simulink model "freego_contact"  (Simulink 8.8)
settings: Solver=ode15s  StartTime=0.0  StopTime=30  MaxStep=0.04  MinStep=1e-10  RelTol=1e-3  EnableMultiTasking=on
model workspace (MATLAB code in the model file):
  | model = quadruped_robot();
undefined symbols (not defined in the file or in its folder): abad_InitAngle, Fpt, freego, gcontact, gcPosVel, hip_InitAngle, knee_InitAngle, quadruped_robot
libraries: simulink x9
settings Model: Creator=roy  LastModifiedBy=LZ
settings DataIOCC: LimitDataPoints=off
settings OptimizationCC: ExpressionDepthLimit=2147483647  InitFltsAndDblsToZero=on
settings DebuggingCC: SolverPrmCheckMsg=warning
settings GRTTargetCC: GeneratePreprocessorConditionals=Use local settings

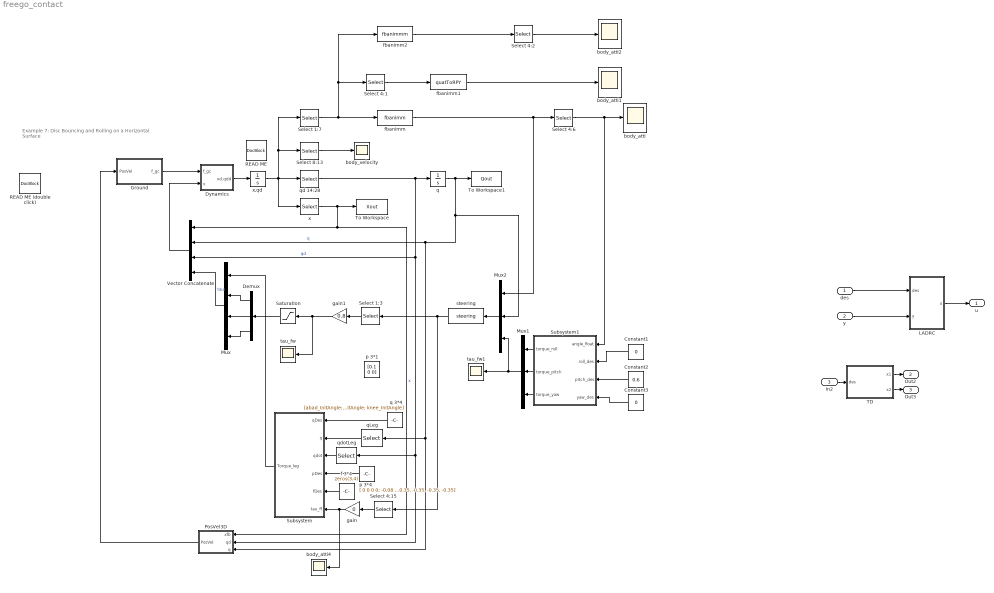
== system freego_contact ==
  note: Example 7: Disc Bouncing and Rolling
      | on a Horizontal Surface
  des : Inport
  y : Inport  Port=2
  In2 : Inport  Port=3
  Constant1 : Constant  Value=0
  Constant2 : Constant  Value=0.6
  Constant3 : Constant  Value=0
  Demux : Demux  Outputs=3
  Dynamics : Subsystem
  Ground : Subsystem
  LADRC : Subsystem
  Mux : Mux
  Mux1 : Mux  Inputs=3
  Mux2 : Mux  Inputs=3
  PosVel3D : Subsystem
  READ ME : simulink/Model-Wide Utilities/DocBlock  DocumentType=Text
      content=|
      | This subsystem builds upon the dynamics calculation in Example 4
      | (free-floating single rigid body).  The two new elements here are: a new
      | argument (f_gc) input to the dynamics calculation, and a new subsystem to
      | calculate the positions and velocities of the ground-contact points.
      |
      | Inside the "Dynamics" subsystem you will find that the floating-base state
      | vector, x, has been combined with the constant npoly and the matrix of
      | ground-contact forces, f_gc.  npoly is required as an argument to
      | rollingdisc.  The reason why it has to be supplied as an input like this
      | is because the executable expression in a "MATLAB Function" block does not
      | have access to the Simulink model's workspace (which is where npoly is
      | defined), so the symbol "npoly" cannot appear directly in this
      | expression.  f_gc is a 6x(npt) matrix, where npt is the number of points
      | defined in the rolling disc model, such that f_gc(:,i) is the spatial
      | force acting on point number i.  The "reshape" block converts it to a
      | column vector such that the first column of f_gc appears in the first six
      | elements, the second column in the next six elements, and so on.  The
      | function gcFD (appearing inside the "MATLAB Function" block) converts this
      | data into the cell-array format required by the f_ext arguments of the
      | dynamics functions, and calls FDfb to calculate the floating-base forward
      | dynamics of the rolling disc.
      |
      | Inside the "PosVel3D" subsystem, you will find the call to gcPosVel.  Once
      | again, npoly is supplied as a constant input, because it is needed as an
      | argument to rollingdisc but cannot appear explicitly in the executable
      | expression in the "MATLAB Function" block.  This function calculates a
      | 6x(npt) matrix such that column i contains the position (first three
      | elements) and velocity (last three elements) of point number i, both
      | expressed in base (body 0) coordinates.
      |
      | This dynamics subsystem can easily be adapted to fixed-base system models,
      | to floating-base models with more than one body, and to system models
      | based on planar arithmetic.  In the case of planar arithmetic, the
      | incoming f_gc is a 3x(npt) matrix whose columns are planar force vectors,
      | and the matrix calculated by gcPosVel is a 4x(npt) matrix containing two
      | 2D vectors in each column.  If vectors of joint position and velocity
      | variables (q and qd) are required instead of or in addition to x, then
      | these must be supplied as inputs to both gcFD and gcPosVel; so you will
      | have to add extra input ports to the blocks "Dynamics" and "PosVel3D".
  READ ME (double click) : simulink/Model-Wide Utilities/DocBlock  DocumentType=Text
  Saturation : Saturate  UpperLimit=3  LowerLimit=-3
  Select 1:3 : Selector  InputPortWidth=15  IndexOptions=Index vector (dialog)  Indices=[1:3]  OutputSizes=1
  Select 1:7 : Selector  InputPortWidth=13+15  IndexOptions=Index vector (dialog)  Indices=[1:7]  OutputSizes=1
  Select 4:1 : Selector  InputPortWidth=7  IndexOptions=Index vector (dialog)  Indices=[1:4]  OutputSizes=1
  Select 4:15 : Selector  InputPortWidth=15  IndexOptions=Index vector (dialog)  Indices=[4:15]  OutputSizes=1
  Select 4:2 : Selector  InputPortWidth=6  IndexOptions=Index vector (dialog)  Indices=[4:6]  OutputSizes=1
  Select 4:6 : Selector  InputPortWidth=6  IndexOptions=Index vector (dialog)  Indices=[4:6]  OutputSizes=1
  Select 8:13 : Selector  InputPortWidth=13+15  IndexOptions=Index vector (dialog)  Indices=[8 9 10 11 12 13]  OutputSizes=1
  Subsystem : Subsystem
  Subsystem1 : Subsystem
  TD : Subsystem
  To Workspace : ToWorkspace  VariableName=Xout  SampleTime=-1
  To Workspace1 : ToWorkspace  VariableName=Qout  SampleTime=-1
  Vector Concatenate : Concatenate  NumInputs=4
  body_atti{,1..2,4} (4 alike) : Scope
  body_velocity : Scope
  f 3*4 : Constant  Value=zeros(3,4)
  fbanimm : MATLABFcn  MATLABFcn=fbanimm  OutputDimensions=6
  fbanimm1 : MATLABFcn  MATLABFcn=quatToRPY  OutputDimensions=3
  fbanimm2 : MATLABFcn  MATLABFcn=fbanimmm  OutputDimensions=6
  gain : Gain  Gain=0
  gain1 : Gain  Gain=0.8
  p 3*1 : Constant  Value=[0.1 0 0]
  p 3*4 : Constant  Value=[ 0 0 0 0; -0.08 0.08 -0.08 0.08; -0.35, -0.35, -0.35, -0.35]
  q : Integrator  InitialCondition=[freego.q_init]'
  q 3*4 : Constant  Value=[abad_InitAngle; hip_InitAngle; knee_InitAngle]
  qLeg : Selector  InputPortWidth=15  IndexOptions=Index vector (dialog)  Indices=[1:12]  OutputSizes=1
  qd 14:28 : Selector  InputPortWidth=13+15  IndexOptions=Index vector (dialog)  Indices=[14:13+15]  OutputSizes=1
  qdotLeg : Selector  InputPortWidth=15  IndexOptions=Index vector (dialog)  Indices=[1:12]  OutputSizes=1
  steering : MATLABFcn  MATLABFcn=steering  OutputDimensions=15  Output1D=off
  tau_fw : Scope
  tau_fw1 : Scope
  x : Selector  InputPortWidth=13+15  IndexOptions=Index vector (dialog)  Indices=[1:13]  OutputSizes=1
  x,qd : Integrator  InitialCondition=[freego.QuatBody, freego.COMLocation, zeros(1,6), zeros(1,15)]'
  u : Outport
  Out2 : Outport  Port=2
  Out3 : Outport  Port=3
  wires:
  PosVel3D/1(PosVel) -> Ground/1(PosVel)
  Dynamics/1(xd,qdd) -> x,qd/1
  x,qd/1 -> x/1, qd 14:28/1, Select 1:7/1, Select 8:13/1
  Select 8:13/1 -> body_velocity/1
  qd 14:28/1 -> q/1, PosVel3D/2(qd), qdotLeg/1, Vector Concatenate/3  "qd"
  q/1 -> To Workspace1/1, Mux2/2, Vector Concatenate/2, PosVel3D/3(q), qLeg/1  "q"
  x/1 -> To Workspace/1, Vector Concatenate/1, PosVel3D/1(xfb)  "x"
  Vector Concatenate/1 -> Dynamics/2(x)
  Ground/1(f_gc) -> Dynamics/1(f_gc)
  Mux/1 -> Vector Concatenate/4  "tau"
  des/1 -> LADRC/1(des)
  y/1 -> LADRC/2(y)
  LADRC/1(u) -> u/1
  In2/1 -> TD/1(des)
  TD/2(x2) -> Out3/1
  TD/1(x1) -> Out2/1
  Demux/1 -> Mux/2
  q 3*4/1 -> Subsystem/1(qDes)
  Subsystem/1(Torque_leg) -> Mux/1
  p 3*4/1 -> Subsystem/4(pDes)
  f 3*4/1 -> Subsystem/5(fDes)
  qLeg/1 -> Subsystem/2(q)
  qdotLeg/1 -> Subsystem/3(qdot)
  Demux/3 -> Mux/4
  Select 1:7/1 -> fbanimm2/1, Select 4:1/1, fbanimm/1
  fbanimm/1 -> Mux2/1, Select 4:6/1
  Select 4:6/1 -> body_atti/1, Subsystem1/1(angle_float)
  Constant2/1 -> Subsystem1/3(pitch_des)
  Subsystem1/1(torque_roll) -> Mux1/1
  Subsystem1/2(torque_pitch) -> Mux1/2
  Subsystem1/3(torque_yaw) -> Mux1/3
  Mux2/1 -> steering/1
  Mux1/1 -> Mux2/3, tau_fw1/1
  steering/1 -> Select 4:15/1, Select 1:3/1
  Demux/2 -> Mux/3
  gain1/1 -> tau_fw/1, Saturation/1
  Select 4:15/1 -> gain/1
  Constant1/1 -> Subsystem1/2(roll_des)
  Constant3/1 -> Subsystem1/4(yaw_des)
  gain/1 -> Subsystem/6(tau_ff), body_atti4/1
  Saturation/1 -> Demux/1
  Select 4:1/1 -> fbanimm1/1
  fbanimm1/1 -> body_atti1/1
  fbanimm2/1 -> Select 4:2/1
  Select 4:2/1 -> body_atti2/1
  Select 1:3/1 -> gain1/1

== system freego_contact/Dynamics ==
  f_gc : Inport
  x : Inport  Port=2
  Quadruped_robot  Dynamics : MATLABFcn  MATLABFcn=gcFD( quadruped_robot, @FDfb, u )  OutputDimensions=[13+15 1]  OutputSignalType=real  Output1D=off
  Reshape : Reshape  OutputDimensionality=Column vector (2-D)
  Vector Concatenate : Concatenate
  xd,qdd : Outport
  wires:
  Vector Concatenate/1 -> Quadruped_robot  Dynamics/1
  Quadruped_robot  Dynamics/1 -> xd,qdd/1
  f_gc/1 -> Reshape/1
  x/1 -> Vector Concatenate/1
  Reshape/1 -> Vector Concatenate/2

== system freego_contact/Ground ==
  PosVel : Inport
  3D Ground Contact : Subsystem  mask(3D Nonlinear Ground Contact with Friction){K=1e6, D=2000, mu=0.1, np=16}
      mask prompts: K "Stiffness (K)"; D "Damping (D)"; mu "Coefficient of Friction (mu)"; np "Number of Contact Points"
      mask help:
      | Given two 3xnp arrays containing contact-point positions and
      | velocities, calculate the 3xnp array of ground-reaction forces
      | acting on those points. Also calculate 1xnp boolean vectors
      | in_ctact (true if normal force >0) and sticking (true if inside
      | or on boundary of friction cone).  Zero-crossing detection is
      | enabled at both make/break contact and stick/slip transitions.
  READ ME : simulink/Model-Wide Utilities/DocBlock  DocumentType=Text
  Terminator : Terminator
  Terminator1 : Terminator
  convert 3D to spatial forces : Subsystem
  select pos : Selector  NumberOfDimensions=2  InputPortWidth=3  IndexOptions=Index vector (dialog),Select all  Indices=[1 2 3],1  OutputSizes=1,1
  select vel : Selector  NumberOfDimensions=2  InputPortWidth=3  IndexOptions=Index vector (dialog),Select all  Indices=[4 5 6],1  OutputSizes=1,1
  f_gc : Outport
  wires:
  PosVel/1 -> select pos/1, select vel/1
  select pos/1 -> convert 3D to spatial forces/1(pos), 3D Ground Contact/1(pos)
  convert 3D to spatial forces/1(force6D) -> f_gc/1
  select vel/1 -> 3D Ground Contact/2(vel)
  3D Ground Contact/1(force) -> convert 3D to spatial forces/2(force3D)
  3D Ground Contact/2(in_ctact) -> Terminator/1
  3D Ground Contact/3(sticking) -> Terminator1/1

== system freego_contact/LADRC ==
  des : Inport
  y : Inport  Port=2
  1/b0 : Gain
  LESO3 : Subsystem
  PID Controller : simulink/Continuous/PID Controller  Controller=PID  TimeDomain=Continuous-time  SampleTime=-1  IntegratorMethod=Forward Euler  FilterMethod=Forward Euler  Form=Parallel  UseFilter=on  ControllerParametersSource=internal  P=10  I=0.01  D=1  N=100  InitialConditionSource=internal  InitialConditionForIntegrator=0  InitialConditionForFilter=0  ExternalReset=none  LimitOutput=off  UpperSaturationLimit=inf  LowerSaturationLimit=-inf  LinearizeAsGain=on  AntiWindupMode=none  Kb=1  TrackingMode=off  Kt=1  PParamMin=[]  PParamMax=[]  IParamMin=[]  IParamMax=[]  DParamMin=[]  DParamMax=[]  NParamMin=[]  NParamMax=[]  KbParamMin=[]  KbParamMax=[]  KtParamMin=[]  KtParamMax=[]  POutMin=[]  POutMax=[]  IOutMin=[]  IOutMax=[]  DOutMin=[]  DOutMax=[]  NOutMin=[]  NOutMax=[]  KbOutMin=[]  KbOutMax=[]  KtOutMin=[]  KtOutMax=[]  IntegratorOutMin=[]  IntegratorOutMax=[]  FilterOutMin=[]  FilterOutMax=[]  SumOutMin=[]  SumOutMax=[]  SumI1OutMin=[]  SumI1OutMax=[]  SumI2OutMin=[]  SumI2OutMax=[]  SumI3OutMin=[]  SumI3OutMax=[]  SumDOutMin=[]  SumDOutMax=[]  SaturationOutMin=[]  SaturationOutMax=[]  IntegratorContinuousStateAttributes=''  IntegratorStateMustResolveToSignalObject=off  IntegratorRTWStateStorageClass=Auto  FilterContinuousStateAttributes=''  FilterStateMustResolveToSignalObject=off  FilterRTWStateStorageClass=Auto  DifferentiatorICPrevScaledInput=0  DifferentiatorOutMin=[]  DifferentiatorOutMax=[]
  PID Controller1 : simulink/Continuous/PID Controller  Controller=PID  TimeDomain=Continuous-time  SampleTime=-1  IntegratorMethod=Forward Euler  FilterMethod=Forward Euler  Form=Parallel  UseFilter=on  ControllerParametersSource=internal  P=10  I=0.01  D=1  N=100  InitialConditionSource=internal  InitialConditionForIntegrator=0  InitialConditionForFilter=0  ExternalReset=none  LimitOutput=off  UpperSaturationLimit=inf  LowerSaturationLimit=-inf  LinearizeAsGain=on  AntiWindupMode=none  Kb=1  TrackingMode=off  Kt=1  PParamMin=[]  PParamMax=[]  IParamMin=[]  IParamMax=[]  DParamMin=[]  DParamMax=[]  NParamMin=[]  NParamMax=[]  KbParamMin=[]  KbParamMax=[]  KtParamMin=[]  KtParamMax=[]  POutMin=[]  POutMax=[]  IOutMin=[]  IOutMax=[]  DOutMin=[]  DOutMax=[]  NOutMin=[]  NOutMax=[]  KbOutMin=[]  KbOutMax=[]  KtOutMin=[]  KtOutMax=[]  IntegratorOutMin=[]  IntegratorOutMax=[]  FilterOutMin=[]  FilterOutMax=[]  SumOutMin=[]  SumOutMax=[]  SumI1OutMin=[]  SumI1OutMax=[]  SumI2OutMin=[]  SumI2OutMax=[]  SumI3OutMin=[]  SumI3OutMax=[]  SumDOutMin=[]  SumDOutMax=[]  SaturationOutMin=[]  SaturationOutMax=[]  IntegratorContinuousStateAttributes=''  IntegratorStateMustResolveToSignalObject=off  IntegratorRTWStateStorageClass=Auto  FilterContinuousStateAttributes=''  FilterStateMustResolveToSignalObject=off  FilterRTWStateStorageClass=Auto  DifferentiatorICPrevScaledInput=0  DifferentiatorOutMin=[]  DifferentiatorOutMax=[]
  Sum1 : Sum  Inputs=|+-
  Sum2 : Sum  Inputs=|+-
  Sum3 : Sum  Inputs=+|+
  Sum4 : Sum  Inputs=|+-
  "TD3 " : Subsystem
  b0 : Gain
  u : Outport
  wires:
  des/1 -> "TD3 "/1(des)
  Sum3/1 -> Sum4/1
  1/b0/1 -> Sum4/2
  PID Controller1/1 -> Sum3/2
  y/1 -> LESO3/1(y)
  Sum2/1 -> PID Controller1/1
  LESO3/3(z3) -> 1/b0/1
  PID Controller/1 -> Sum3/1
  "TD3 "/2(x2) -> Sum2/1
  LESO3/2(z2) -> Sum2/2
  "TD3 "/1(x1) -> Sum1/1
  Sum1/1 -> PID Controller/1
  b0/1 -> LESO3/2(b0u)
  LESO3/1(z1) -> Sum1/2
  Sum4/1 -> u/1, b0/1

== system freego_contact/PosVel3D ==
  note: The constant supplies the
      | argument for rollingdisc
  xfb : Inport
  qd : Inport  Port=2
  q : Inport  Port=3
  Vector Concatenate1 : Concatenate  NumInputs=3
  gcPosVel : MATLABFcn  MATLABFcn=gcPosVel( quadruped_robot(), u(1:13), u(14:28), u(29:43))  OutputDimensions=[6 16]  OutputSignalType=real  Output1D=off
  PosVel : Outport
  wires:
  gcPosVel/1 -> PosVel/1
  Vector Concatenate1/1 -> gcPosVel/1
  q/1 -> Vector Concatenate1/2
  xfb/1 -> Vector Concatenate1/1
  qd/1 -> Vector Concatenate1/3

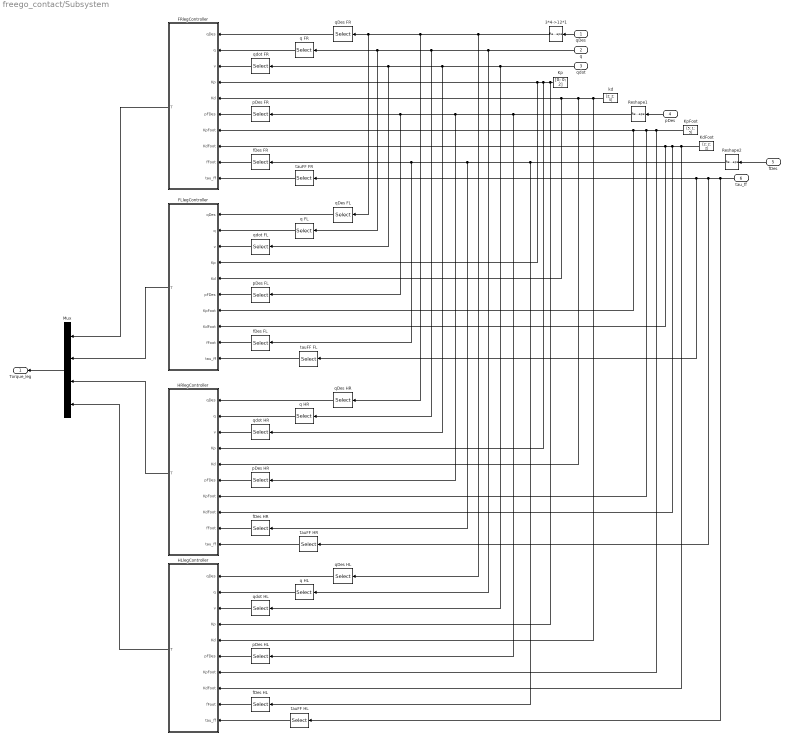
== system freego_contact/Subsystem ==
  qDes : Inport
  q : Inport  Port=2
  qdot : Inport  Port=3
  pDes : Inport  Port=4
  fDes : Inport  Port=5
  tau_ff : Inport  Port=6
  3*4->12*1 : Reshape  OutputDimensionality=Column vector (2-D)
  FLlegController : Subsystem
  FRlegController : Subsystem
  HLlegController : Subsystem
  HRlegController : Subsystem
  KdFoot : Constant  Value=[2; 2; 2]
  Kp : Constant  Value=[0; 0; 2]
  KpFoot : Constant  Value=[5; 1; 5]
  Mux : Mux
  Reshape1 : Reshape  OutputDimensionality=Column vector (2-D)
  Reshape2 : Reshape  OutputDimensionality=Column vector (2-D)
  fDes FL : Selector  InputPortWidth=12  IndexOptions=Index vector (dialog)  Indices=[4:6]  OutputSizes=1
  fDes FR : Selector  InputPortWidth=12  IndexOptions=Index vector (dialog)  Indices=[1:3]  OutputSizes=1
  fDes HL : Selector  InputPortWidth=12  IndexOptions=Index vector (dialog)  Indices=[10:12]  OutputSizes=1
  fDes HR : Selector  InputPortWidth=12  IndexOptions=Index vector (dialog)  Indices=[7:9]  OutputSizes=1
  kd : Constant  Value=[2; 2; 5]
  pDes FL : Selector  InputPortWidth=12  IndexOptions=Index vector (dialog)  Indices=[4:6]  OutputSizes=1
  pDes FR : Selector  InputPortWidth=12  IndexOptions=Index vector (dialog)  Indices=[1:3]  OutputSizes=1
  pDes HL : Selector  InputPortWidth=12  IndexOptions=Index vector (dialog)  Indices=[10:12]  OutputSizes=1
  pDes HR : Selector  InputPortWidth=12  IndexOptions=Index vector (dialog)  Indices=[7:9]  OutputSizes=1
  q FL : Selector  InputPortWidth=12  IndexOptions=Index vector (dialog)  Indices=[4:6]  OutputSizes=1
  q FR : Selector  InputPortWidth=12  IndexOptions=Index vector (dialog)  Indices=[1:3]  OutputSizes=1
  q HL : Selector  InputPortWidth=12  IndexOptions=Index vector (dialog)  Indices=[10:12]  OutputSizes=1
  q HR : Selector  InputPortWidth=12  IndexOptions=Index vector (dialog)  Indices=[7:9]  OutputSizes=1
  qDes FL : Selector  InputPortWidth=12  IndexOptions=Index vector (dialog)  Indices=[4:6]  OutputSizes=1
  qDes FR : Selector  InputPortWidth=12  IndexOptions=Index vector (dialog)  Indices=[1:3]  OutputSizes=1
  qDes HL : Selector  InputPortWidth=12  IndexOptions=Index vector (dialog)  Indices=[10:12]  OutputSizes=1
  qDes HR : Selector  InputPortWidth=12  IndexOptions=Index vector (dialog)  Indices=[7:9]  OutputSizes=1
  qdot FL : Selector  InputPortWidth=12  IndexOptions=Index vector (dialog)  Indices=[4:6]  OutputSizes=1
  qdot FR : Selector  InputPortWidth=12  IndexOptions=Index vector (dialog)  Indices=[1:3]  OutputSizes=1
  qdot HL : Selector  InputPortWidth=12  IndexOptions=Index vector (dialog)  Indices=[10:12]  OutputSizes=1
  qdot HR : Selector  InputPortWidth=12  IndexOptions=Index vector (dialog)  Indices=[7:9]  OutputSizes=1
  tauFF FL : Selector  InputPortWidth=12  IndexOptions=Index vector (dialog)  Indices=[4:6]  OutputSizes=1
  tauFF FR : Selector  InputPortWidth=12  IndexOptions=Index vector (dialog)  Indices=[1:3]  OutputSizes=1
  tauFF HL : Selector  InputPortWidth=12  IndexOptions=Index vector (dialog)  Indices=[10:12]  OutputSizes=1
  tauFF HR : Selector  InputPortWidth=12  IndexOptions=Index vector (dialog)  Indices=[7:9]  OutputSizes=1
  Torque_leg : Outport
  wires:
  q FR/1 -> FRlegController/2(q)
  qDes/1 -> 3*4->12*1/1
  pDes/1 -> Reshape1/1
  qdot/1 -> qdot HR/1, qdot FL/1, qdot FR/1, qdot HL/1
  qdot FR/1 -> FRlegController/3(v)
  q FL/1 -> FLlegController/2(q)
  kd/1 -> HLlegController/5(Kd), HRlegController/5(Kd), FLlegController/5(Kd), FRlegController/5(Kd)
  KpFoot/1 -> FRlegController/7(KpFoot), FLlegController/7(KpFoot), HRlegController/7(KpFoot), HLlegController/7(KpFoot)
  qDes FL/1 -> FLlegController/1(qDes)
  pDes FL/1 -> FLlegController/6(pFDes)
  q/1 -> q HR/1, q FL/1, q FR/1, q HL/1
  qdot FL/1 -> FLlegController/3(v)
  qDes FR/1 -> FRlegController/1(qDes)
  pDes FR/1 -> FRlegController/6(pFDes)
  3*4->12*1/1 -> qDes HR/1, qDes FL/1, qDes FR/1, qDes HL/1
  Reshape1/1 -> pDes HR/1, pDes FL/1, pDes FR/1, pDes HL/1
  q HR/1 -> HRlegController/2(q)
  qDes HR/1 -> HRlegController/1(qDes)
  pDes HR/1 -> HRlegController/6(pFDes)
  qdot HR/1 -> HRlegController/3(v)
  q HL/1 -> HLlegController/2(q)
  Kp/1 -> HLlegController/4(Kp), HRlegController/4(Kp), FLlegController/4(Kp), FRlegController/4(Kp)
  KdFoot/1 -> FRlegController/8(KdFoot), FLlegController/8(KdFoot), HRlegController/8(KdFoot), HLlegController/8(KdFoot)
  Reshape2/1 -> fDes HL/1, fDes HR/1, fDes FL/1, fDes FR/1
  qDes HL/1 -> HLlegController/1(qDes)
  pDes HL/1 -> HLlegController/6(pFDes)
  qdot HL/1 -> HLlegController/3(v)
  Mux/1 -> Torque_leg/1
  FRlegController/1(T) -> Mux/1
  FLlegController/1(T) -> Mux/2
  HRlegController/1(T) -> Mux/3
  HLlegController/1(T) -> Mux/4
  fDes/1 -> Reshape2/1
  fDes FR/1 -> FRlegController/9(fFoot)
  fDes FL/1 -> FLlegController/9(fFoot)
  fDes HR/1 -> HRlegController/9(fFoot)
  fDes HL/1 -> HLlegController/9(fFoot)
  tauFF FL/1 -> FLlegController/10(tau_ff)
  tauFF HR/1 -> HRlegController/10(tau_ff)
  tauFF HL/1 -> HLlegController/10(tau_ff)
  tauFF FR/1 -> FRlegController/10(tau_ff)
  tau_ff/1 -> tauFF HL/1, tauFF HR/1, tauFF FL/1, tauFF FR/1

== system freego_contact/Subsystem1 ==
  angle_float : Inport
  roll_des : Inport  Port=2
  pitch_des : Inport  Port=3
  yaw_des : Inport  Port=4
  Demux : Demux  Outputs=3
  LADRC_Pitch : Subsystem
  LADRC_Roll : Subsystem
  LADRC_Yaw : Subsystem
  p : Gain  Gain=0
  p1 : Gain  Gain=-1
  p2 : Gain  Gain=0
  torque_roll : Outport
  torque_pitch : Outport  Port=2
  torque_yaw : Outport  Port=3
  wires:
  LADRC_Yaw/1(u) -> p2/1
  yaw_des/1 -> LADRC_Yaw/1(des)
  pitch_des/1 -> LADRC_Pitch/1(des)
  LADRC_Pitch/1(u) -> p1/1
  angle_float/1 -> Demux/1
  p/1 -> torque_roll/1
  roll_des/1 -> LADRC_Roll/1(des)
  LADRC_Roll/1(u) -> p/1
  Demux/2 -> LADRC_Pitch/2(y)
  Demux/1 -> LADRC_Roll/2(y)
  Demux/3 -> LADRC_Yaw/2(y)
  p1/1 -> torque_pitch/1
  p2/1 -> torque_yaw/1

== system freego_contact/TD ==
  des : Inport
  MATLAB Function1 : MATLAB Function  TreatAsAtomicUnit=on
  Product : Product
  Product1 : Product
  Sum : Sum  Inputs=+-|
  h : Constant
  r : Constant  Value=10000000000000000000000000
  sx1 : Integrator
  sx2 : Integrator
  x1 : Outport
  x2 : Outport  Port=2
  wires:
  sx2/1 -> MATLAB Function1/2(x2), x2/1, Product1/1
  h/1 -> MATLAB Function1/4(h), Product/2, Product1/2  "h"
  Product/1 -> sx2/1
  MATLAB Function1/1(fh) -> Product/1
  sx1/1 -> Sum/1, x1/1
  r/1 -> MATLAB Function1/3(r)
  Product1/1 -> sx1/1
  Sum/1 -> MATLAB Function1/1(x1)
  des/1 -> Sum/2

== system freego_contact/Ground/3D Ground Contact ==
  pos : Inport
  vel : Inport  Port=2
  Compare To Constant : simulink/Logic and Bit Operations/Compare To Constant  relop=<=  const=1  OutDataTypeStr=boolean
  Compare To Zero : simulink/Logic and Bit Operations/Compare To Zero  relop=>  OutDataTypeStr=boolean
  K,D,mu : Constant  Value=[ [K; D; mu] zeros(3,np-1) ]  VectorParams1D=off
  READ ME : simulink/Model-Wide Utilities/DocBlock  DocumentType=Text
      content=|
      | The constant block supplies the parameters K, D and mu to the function
      | gcontact.  This is necessary because K, D and mu are defined in the
      | workspace of this particular masked subsystem, but the executable
      | expression in the "MATLAB Function" block does not have access to this
      | workspace, so the symbols K, D and mu cannot appear directly in the
      | executable expression.
      |
      | The ">0" block and the "<=1" block both have zero-crossing enabled.  The
      | former detects transitions between contact and non-contact, whereas the
      | latter detects transitions between sticking (due to friction) and
      | slipping.  A point can be sticking only if it is also in contact.  A
      | zero-crossing event occurs whenever any one point makes a transition.
      |
      | The state variable, u, is a 2x(np) matrix containing the horizontal
      | component of the local ground deformation for each point.  This quantity
      | is used to calculate the tangential (i.e., frictional) component of the
      | ground reaction force.
      |
      | When a point loses contact, its associated state variable, u(:,i), decays
      | to zero with a time constant of D/K.  If this ratio is small then the
      | corresponding differential equation is fast, and it is necessary to use
      | small integration time steps.  For example, if K=1e6 and D=2000 then
      | D/K=0.002 and u(:,i) decays in proportion to exp(-500t).  Increasing K
      | makes the surface stiffer, and decreasing D/K makes it bouncier, but the
      | latter also makes the post-contact recovery faster.  The degree of
      | bounciness depends on the mass of the impacting body: a heavier body will
      | bounce more.
      |
      | To adapt this subsystem to work in 2D, the only things that change are the
      | row dimensions of various matrices.  You will have to alter the row
      | selections in the executable expression in the "MATLAB Function" block,
      | and also the dimensions of its output matrix, and you will have to change
      | the row selections in the various "select" blocks.
      |
      | For more information, see "The Simulink Ground Contact Model" in the
      | spatial_v2 documentation directory.
  Vector Concatenate : Concatenate  NumInputs=4  Mode=Multidimensional array
  gcontact : MATLABFcn  MATLABFcn=gcontact( u(1,1), u(2,1), u(3,1), u(4:6,:), u(7:9,:), u(10:11,:) )  OutputDimensions=[6 np]  OutputSignalType=real  Output1D=off
  select fcone : Selector  NumberOfDimensions=2  InputPortWidth=3  IndexOptions=Index vector (dialog),Select all  Indices=[6],1  OutputSizes=1,1
  select force : Selector  NumberOfDimensions=2  InputPortWidth=3  IndexOptions=Index vector (dialog),Select all  Indices=[1 2 3],1  OutputSizes=1,1
  select fz : Selector  NumberOfDimensions=2  InputPortWidth=3  IndexOptions=Index vector (dialog),Select all  Indices=[3],1  OutputSizes=1,1
  select ud : Selector  NumberOfDimensions=2  InputPortWidth=3  IndexOptions=Index vector (dialog),Select all  Indices=[4 5],1  OutputSizes=1,1
  u : Integrator
  force : Outport
  in_ctact : Outport  Port=2
  sticking : Outport  Port=3
  wires:
  Vector Concatenate/1 -> gcontact/1
  select ud/1 -> u/1
  gcontact/1 -> select fz/1, select ud/1, select fcone/1, select force/1
  select force/1 -> force/1
  select fz/1 -> Compare To Zero/1
  Compare To Zero/1 -> in_ctact/1
  select fcone/1 -> Compare To Constant/1
  Compare To Constant/1 -> sticking/1
  u/1 -> Vector Concatenate/4
  vel/1 -> Vector Concatenate/3
  pos/1 -> Vector Concatenate/2
  K,D,mu/1 -> Vector Concatenate/1

== system freego_contact/Ground/convert 3D to spatial forces ==
  note: calculate a 6*npt matrix of spatial force vectors (one per column)
      | from a 3*npt matrix of position vectors specifying the points
      | through which the forces act, and a 3*npt matrix of force vectors
  pos : Inport
  force3D : Inport  Port=2
  Fpt : MATLABFcn  MATLABFcn=Fpt( u(4:6,:), u(1:3,:) )  OutputSignalType=real  Output1D=off
  Matrix Concatenate : Concatenate  Mode=Multidimensional array
  force6D : Outport
  wires:
  force3D/1 -> Matrix Concatenate/2
  pos/1 -> Matrix Concatenate/1
  Matrix Concatenate/1 -> Fpt/1
  Fpt/1 -> force6D/1

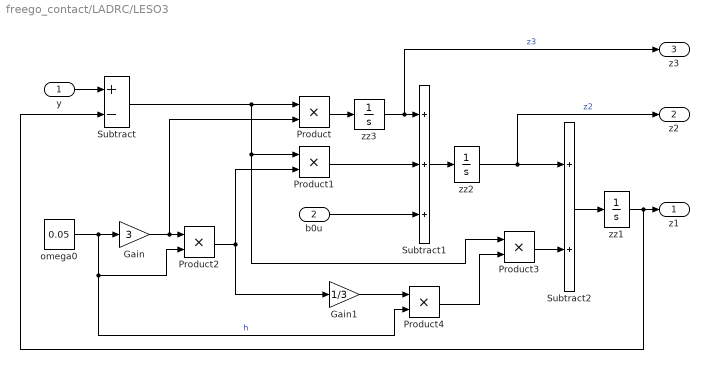
== system freego_contact/LADRC/LESO3 ==
  y : Inport
  b0u : Inport  Port=2
  Gain : Gain  Gain=3
  Gain1 : Gain  Gain=1/3
  Product{,1..4} (5 alike) : Product
  Subtract : Sum  Inputs=+-
  Subtract1 : Sum  Inputs=+++
  Subtract2 : Sum
  omega0 : Constant  Value=0.05
  zz1 : Integrator
  zz2 : Integrator
  zz3 : Integrator
  z1 : Outport
  z2 : Outport  Port=2
  z3 : Outport  Port=3
  wires:
  y/1 -> Subtract/1
  Subtract/1 -> Product/1, Product3/1, Product1/1
  omega0/1 -> Gain/1, Product4/2, Product2/2  "h"
  Gain/1 -> Product/2, Product2/1
  Product/1 -> zz3/1
  zz3/1 -> z3/1, Subtract1/1  "z3"
  b0u/1 -> Subtract1/3
  Product1/1 -> Subtract1/2
  Product2/1 -> Gain1/1, Product1/2
  Subtract1/1 -> zz2/1
  zz2/1 -> Subtract2/1, z2/1  "z2"
  zz1/1 -> Subtract/2, z1/1
  Product3/1 -> Subtract2/2
  Product4/1 -> Product3/2
  Subtract2/1 -> zz1/1
  Gain1/1 -> Product4/1

== system freego_contact/LADRC/TD3  ==
  des : Inport
  Gain : Gain  Gain=-1
  MATLAB Function1 : MATLAB Function  TreatAsAtomicUnit=on
  Product : Product
  d : Constant  Value=0.05
  r : Constant  Value=300
  sx1 : Integrator
  sx2 : Integrator
  x1 : Outport
  x2 : Outport  Port=2
  wires:
  d/1 -> MATLAB Function1/5(d)  "h"
  Product/1 -> sx2/1
  MATLAB Function1/1(f) -> Product/1
  sx1/1 -> MATLAB Function1/1(x1), x1/1
  r/1 -> Gain/1, MATLAB Function1/4(r)
  sx2/1 -> MATLAB Function1/2(x2), sx1/1, x2/1
  des/1 -> MATLAB Function1/3(u)
  Gain/1 -> Product/2

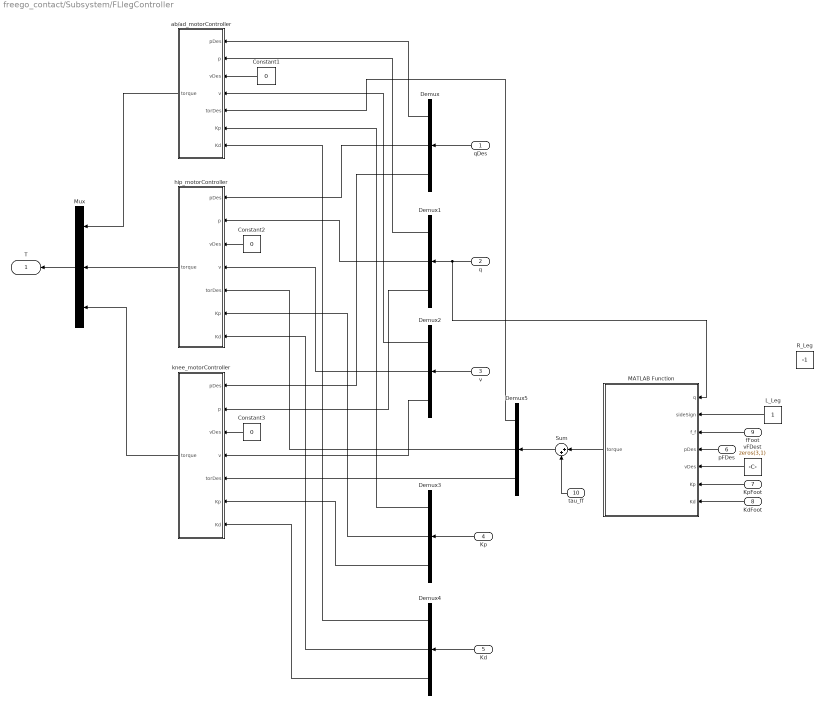
== system freego_contact/Subsystem/FLlegController ==
  qDes : Inport
  q : Inport  Port=2
  v : Inport  Port=3
  Kp : Inport  Port=4
  Kd : Inport  Port=5
  pFDes : Inport  Port=6
  KpFoot : Inport  Port=7
  KdFoot : Inport  Port=8
  fFoot : Inport  Port=9
  tau_ff : Inport  Port=10
  Constant1 : Constant  Value=0
  Constant2 : Constant  Value=0
  Constant3 : Constant  Value=0
  Demux{,1..5} (6 alike) : Demux  Outputs=3
  L_Leg : Constant
  MATLAB Function : MATLAB Function  TreatAsAtomicUnit=on
  Mux : Mux  Inputs=3
  R_Leg : Constant  Value=-1
  Sum : Sum  Inputs=|++
  ab/ad_motorController : Subsystem
  hip_motorController : Subsystem
  knee_motorController : Subsystem
  vFDest : Constant  Value=zeros(3,1)
  T : Outport
  wires:
  Demux/1 -> ab/ad_motorController/1(pDes)
  Demux1/1 -> ab/ad_motorController/2(p)
  Demux2/1 -> ab/ad_motorController/4(v)
  Demux3/1 -> ab/ad_motorController/6(Kp)
  Demux5/1 -> ab/ad_motorController/5(torDes)
  Constant1/1 -> ab/ad_motorController/3(vDes)
  Demux4/1 -> ab/ad_motorController/7(Kd)
  ab/ad_motorController/1(torque) -> Mux/1
  Constant2/1 -> hip_motorController/3(vDes)
  Demux2/2 -> hip_motorController/4(v)
  Demux/2 -> hip_motorController/1(pDes)
  Demux1/3 -> knee_motorController/2(p)
  Demux5/2 -> hip_motorController/5(torDes)
  Demux3/2 -> hip_motorController/6(Kp)
  Demux5/3 -> knee_motorController/5(torDes)
  Demux/3 -> knee_motorController/1(pDes)
  Constant3/1 -> knee_motorController/3(vDes)
  Demux4/2 -> hip_motorController/7(Kd)
  hip_motorController/1(torque) -> Mux/2
  Demux3/3 -> knee_motorController/6(Kp)
  Demux1/2 -> hip_motorController/2(p)
  knee_motorController/1(torque) -> Mux/3
  Demux4/3 -> knee_motorController/7(Kd)
  qDes/1 -> Demux/1
  q/1 -> MATLAB Function/1(q), Demux1/1
  v/1 -> Demux2/1
  Demux2/3 -> knee_motorController/4(v)
  Kp/1 -> Demux3/1
  Kd/1 -> Demux4/1
  Mux/1 -> T/1
  fFoot/1 -> MATLAB Function/3(f_f)
  KdFoot/1 -> MATLAB Function/7(Kd)
  KpFoot/1 -> MATLAB Function/6(Kp)
  vFDest/1 -> MATLAB Function/5(vDes)
  pFDes/1 -> MATLAB Function/4(pDes)
  L_Leg/1 -> MATLAB Function/2(sideSign)
  tau_ff/1 -> Sum/2
  MATLAB Function/1(torque) -> Sum/1
  Sum/1 -> Demux5/1

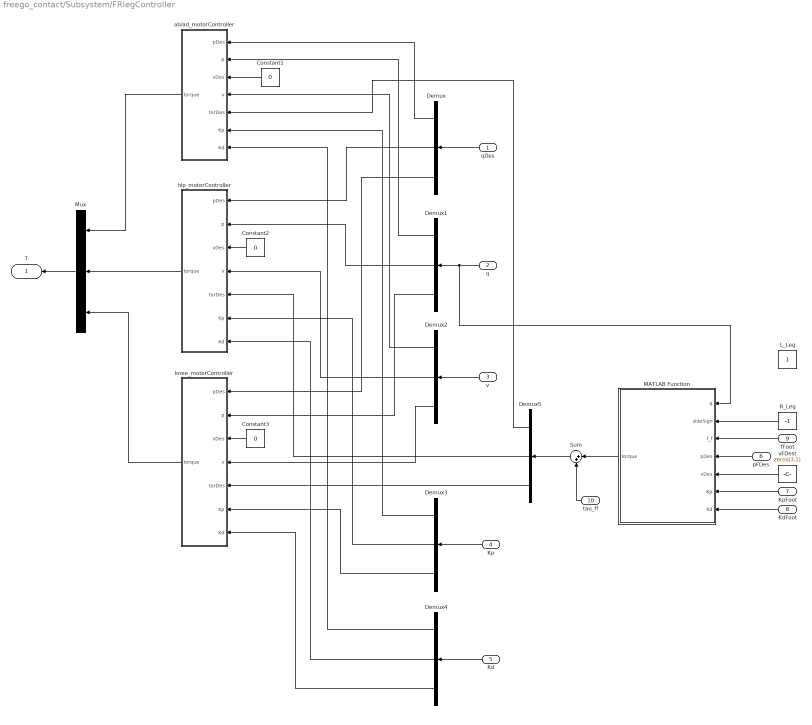
== system freego_contact/Subsystem/FRlegController ==
  qDes : Inport
  q : Inport  Port=2
  v : Inport  Port=3
  Kp : Inport  Port=4
  Kd : Inport  Port=5
  pFDes : Inport  Port=6
  KpFoot : Inport  Port=7
  KdFoot : Inport  Port=8
  fFoot : Inport  Port=9
  tau_ff : Inport  Port=10
  Constant1 : Constant  Value=0
  Constant2 : Constant  Value=0
  Constant3 : Constant  Value=0
  Demux{,1..5} (6 alike) : Demux  Outputs=3
  L_Leg : Constant
  MATLAB Function : MATLAB Function  TreatAsAtomicUnit=on
  Mux : Mux  Inputs=3
  R_Leg : Constant  Value=-1
  Sum : Sum  Inputs=|++
  ab/ad_motorController : Subsystem
  hip_motorController : Subsystem
  knee_motorController : Subsystem
  vFDest : Constant  Value=zeros(3,1)
  T : Outport
  wires:
  Demux/1 -> ab/ad_motorController/1(pDes)
  Demux1/1 -> ab/ad_motorController/2(p)
  Demux2/1 -> ab/ad_motorController/4(v)
  Demux3/1 -> ab/ad_motorController/6(Kp)
  Demux5/1 -> ab/ad_motorController/5(torDes)
  Constant1/1 -> ab/ad_motorController/3(vDes)
  Demux4/1 -> ab/ad_motorController/7(Kd)
  ab/ad_motorController/1(torque) -> Mux/1
  Constant2/1 -> hip_motorController/3(vDes)
  Demux2/2 -> hip_motorController/4(v)
  Demux/2 -> hip_motorController/1(pDes)
  Demux1/3 -> knee_motorController/2(p)
  Demux5/2 -> hip_motorController/5(torDes)
  Demux3/2 -> hip_motorController/6(Kp)
  Demux5/3 -> knee_motorController/5(torDes)
  Demux/3 -> knee_motorController/1(pDes)
  Constant3/1 -> knee_motorController/3(vDes)
  Demux4/2 -> hip_motorController/7(Kd)
  hip_motorController/1(torque) -> Mux/2
  Demux3/3 -> knee_motorController/6(Kp)
  Demux1/2 -> hip_motorController/2(p)
  knee_motorController/1(torque) -> Mux/3
  Demux4/3 -> knee_motorController/7(Kd)
  qDes/1 -> Demux/1
  q/1 -> MATLAB Function/1(q), Demux1/1
  v/1 -> Demux2/1
  Demux2/3 -> knee_motorController/4(v)
  Kp/1 -> Demux3/1
  Kd/1 -> Demux4/1
  Mux/1 -> T/1
  fFoot/1 -> MATLAB Function/3(f_f)
  KdFoot/1 -> MATLAB Function/7(Kd)
  KpFoot/1 -> MATLAB Function/6(Kp)
  vFDest/1 -> MATLAB Function/5(vDes)
  pFDes/1 -> MATLAB Function/4(pDes)
  MATLAB Function/1(torque) -> Sum/1
  R_Leg/1 -> MATLAB Function/2(sideSign)
  tau_ff/1 -> Sum/2
  Sum/1 -> Demux5/1

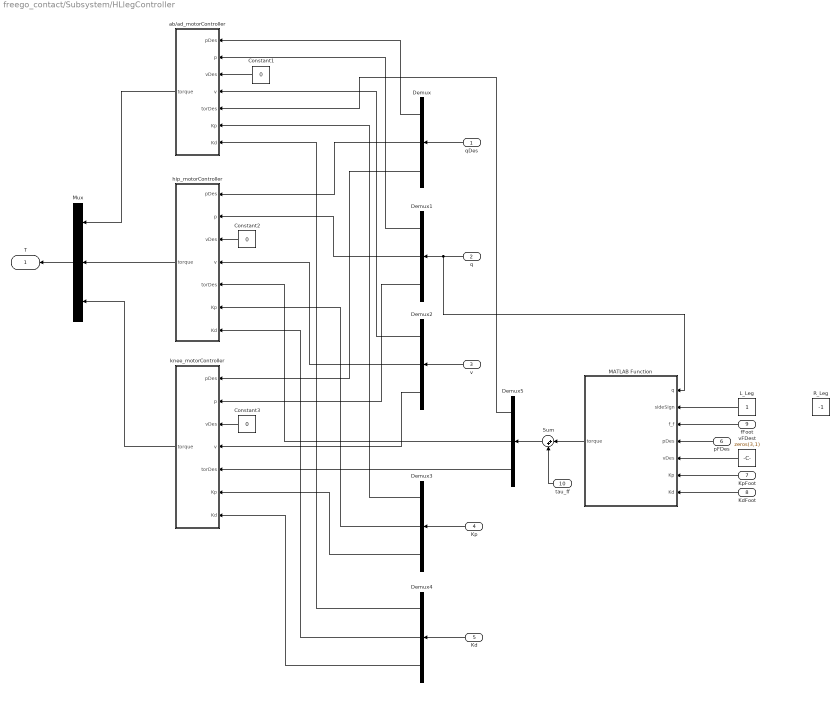
== system freego_contact/Subsystem/HLlegController ==
  qDes : Inport
  q : Inport  Port=2
  v : Inport  Port=3
  Kp : Inport  Port=4
  Kd : Inport  Port=5
  pFDes : Inport  Port=6
  KpFoot : Inport  Port=7
  KdFoot : Inport  Port=8
  fFoot : Inport  Port=9
  tau_ff : Inport  Port=10
  Constant1 : Constant  Value=0
  Constant2 : Constant  Value=0
  Constant3 : Constant  Value=0
  Demux{,1..5} (6 alike) : Demux  Outputs=3
  L_Leg : Constant
  MATLAB Function : MATLAB Function  TreatAsAtomicUnit=on
  Mux : Mux  Inputs=3
  R_Leg : Constant  Value=-1
  Sum : Sum  Inputs=|++
  ab/ad_motorController : Subsystem
  hip_motorController : Subsystem
  knee_motorController : Subsystem
  vFDest : Constant  Value=zeros(3,1)
  T : Outport
  wires:
  Demux/1 -> ab/ad_motorController/1(pDes)
  Demux1/1 -> ab/ad_motorController/2(p)
  Demux2/1 -> ab/ad_motorController/4(v)
  Demux3/1 -> ab/ad_motorController/6(Kp)
  Demux5/1 -> ab/ad_motorController/5(torDes)
  Constant1/1 -> ab/ad_motorController/3(vDes)
  Demux4/1 -> ab/ad_motorController/7(Kd)
  ab/ad_motorController/1(torque) -> Mux/1
  Constant2/1 -> hip_motorController/3(vDes)
  Demux2/2 -> hip_motorController/4(v)
  Demux/2 -> hip_motorController/1(pDes)
  Demux1/3 -> knee_motorController/2(p)
  Demux5/2 -> hip_motorController/5(torDes)
  Demux3/2 -> hip_motorController/6(Kp)
  Demux5/3 -> knee_motorController/5(torDes)
  Demux/3 -> knee_motorController/1(pDes)
  Constant3/1 -> knee_motorController/3(vDes)
  Demux4/2 -> hip_motorController/7(Kd)
  hip_motorController/1(torque) -> Mux/2
  Demux3/3 -> knee_motorController/6(Kp)
  Demux1/2 -> hip_motorController/2(p)
  knee_motorController/1(torque) -> Mux/3
  Demux4/3 -> knee_motorController/7(Kd)
  qDes/1 -> Demux/1
  q/1 -> MATLAB Function/1(q), Demux1/1
  v/1 -> Demux2/1
  Demux2/3 -> knee_motorController/4(v)
  Kp/1 -> Demux3/1
  Kd/1 -> Demux4/1
  Mux/1 -> T/1
  fFoot/1 -> MATLAB Function/3(f_f)
  KdFoot/1 -> MATLAB Function/7(Kd)
  KpFoot/1 -> MATLAB Function/6(Kp)
  vFDest/1 -> MATLAB Function/5(vDes)
  pFDes/1 -> MATLAB Function/4(pDes)
  L_Leg/1 -> MATLAB Function/2(sideSign)
  tau_ff/1 -> Sum/2
  MATLAB Function/1(torque) -> Sum/1
  Sum/1 -> Demux5/1

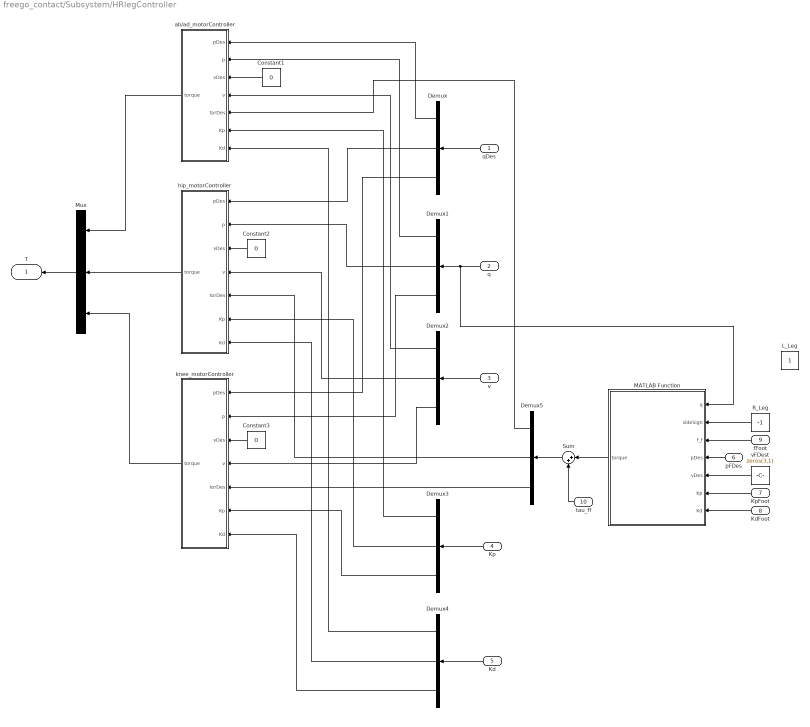
== system freego_contact/Subsystem/HRlegController ==
  qDes : Inport
  q : Inport  Port=2
  v : Inport  Port=3
  Kp : Inport  Port=4
  Kd : Inport  Port=5
  pFDes : Inport  Port=6
  KpFoot : Inport  Port=7
  KdFoot : Inport  Port=8
  fFoot : Inport  Port=9
  tau_ff : Inport  Port=10
  Constant1 : Constant  Value=0
  Constant2 : Constant  Value=0
  Constant3 : Constant  Value=0
  Demux{,1..5} (6 alike) : Demux  Outputs=3
  L_Leg : Constant
  MATLAB Function : MATLAB Function  TreatAsAtomicUnit=on
  Mux : Mux  Inputs=3
  R_Leg : Constant  Value=-1
  Sum : Sum  Inputs=|++
  ab/ad_motorController : Subsystem
  hip_motorController : Subsystem
  knee_motorController : Subsystem
  vFDest : Constant  Value=zeros(3,1)
  T : Outport
  wires:
  Demux/1 -> ab/ad_motorController/1(pDes)
  Demux1/1 -> ab/ad_motorController/2(p)
  Demux2/1 -> ab/ad_motorController/4(v)
  Demux3/1 -> ab/ad_motorController/6(Kp)
  Demux5/1 -> ab/ad_motorController/5(torDes)
  Constant1/1 -> ab/ad_motorController/3(vDes)
  Demux4/1 -> ab/ad_motorController/7(Kd)
  ab/ad_motorController/1(torque) -> Mux/1
  Constant2/1 -> hip_motorController/3(vDes)
  Demux2/2 -> hip_motorController/4(v)
  Demux/2 -> hip_motorController/1(pDes)
  Demux1/3 -> knee_motorController/2(p)
  Demux5/2 -> hip_motorController/5(torDes)
  Demux3/2 -> hip_motorController/6(Kp)
  Demux5/3 -> knee_motorController/5(torDes)
  Demux/3 -> knee_motorController/1(pDes)
  Constant3/1 -> knee_motorController/3(vDes)
  Demux4/2 -> hip_motorController/7(Kd)
  hip_motorController/1(torque) -> Mux/2
  Demux3/3 -> knee_motorController/6(Kp)
  Demux1/2 -> hip_motorController/2(p)
  knee_motorController/1(torque) -> Mux/3
  Demux4/3 -> knee_motorController/7(Kd)
  qDes/1 -> Demux/1
  q/1 -> MATLAB Function/1(q), Demux1/1
  v/1 -> Demux2/1
  Demux2/3 -> knee_motorController/4(v)
  Kp/1 -> Demux3/1
  Kd/1 -> Demux4/1
  Mux/1 -> T/1
  fFoot/1 -> MATLAB Function/3(f_f)
  KdFoot/1 -> MATLAB Function/7(Kd)
  KpFoot/1 -> MATLAB Function/6(Kp)
  vFDest/1 -> MATLAB Function/5(vDes)
  pFDes/1 -> MATLAB Function/4(pDes)
  R_Leg/1 -> MATLAB Function/2(sideSign)
  tau_ff/1 -> Sum/2
  MATLAB Function/1(torque) -> Sum/1
  Sum/1 -> Demux5/1

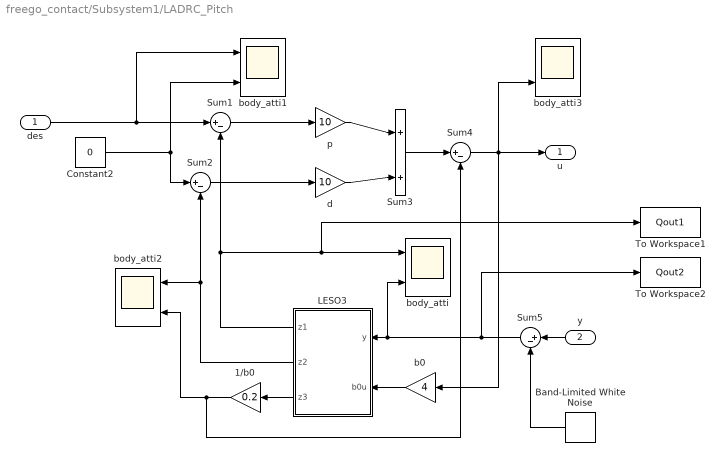
== system freego_contact/Subsystem1/LADRC_Pitch ==
  des : Inport
  y : Inport  Port=2
  1/b0 : Gain  Gain=0.2
  Band-Limited White Noise : simulink/Sources/Band-Limited White Noise  Cov=[0.00001]  Ts=0.05  seed=[23341]
  Constant2 : Constant  Value=0
  LESO3 : Subsystem
  Sum{1..2,4..5} (4 alike) : Sum  Inputs=|+-
  Sum3 : Sum  Inputs=+|+
  To Workspace1 : ToWorkspace  VariableName=Qout1  SampleTime=-1
  To Workspace2 : ToWorkspace  VariableName=Qout2  SampleTime=-1
  b0 : Gain  Gain=4
  body_atti{,1..3} (4 alike) : Scope  NumInputPorts=2
  d : Gain  Gain=10
  p : Gain  Gain=10
  u : Outport
  wires:
  Sum3/1 -> Sum4/1
  1/b0/1 -> Sum4/2, body_atti2/2
  d/1 -> Sum3/2
  Sum2/1 -> d/1
  LESO3/3(z3) -> 1/b0/1
  p/1 -> Sum3/1
  LESO3/2(z2) -> body_atti2/1, Sum2/2
  Sum1/1 -> p/1
  b0/1 -> LESO3/2(b0u)
  LESO3/1(z1) -> To Workspace1/1, body_atti/1, Sum1/2
  Sum4/1 -> u/1, body_atti3/2, b0/1
  des/1 -> Sum1/1, body_atti1/1
  Constant2/1 -> Sum2/1, body_atti1/2
  Sum5/1 -> To Workspace2/1, body_atti/2, LESO3/1(y)
  y/1 -> Sum5/1
  Band-Limited White Noise/1 -> Sum5/2

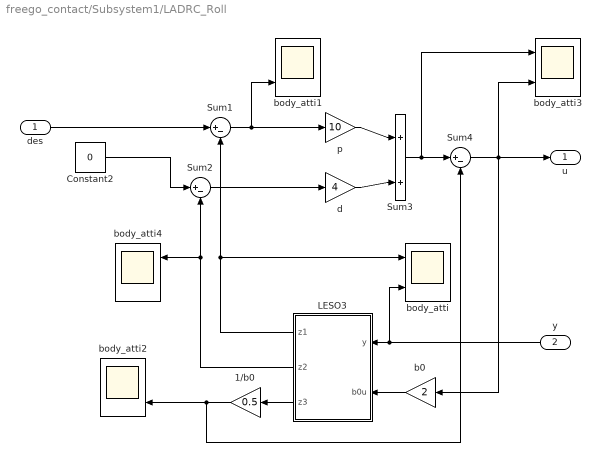
== system freego_contact/Subsystem1/LADRC_Roll ==
  des : Inport
  y : Inport  Port=2
  1/b0 : Gain  Gain=0.5
  Constant2 : Constant  Value=0
  LESO3 : Subsystem
  Sum1 : Sum  Inputs=|+-
  Sum2 : Sum  Inputs=|+-
  Sum3 : Sum  Inputs=+|+
  Sum4 : Sum  Inputs=|+-
  b0 : Gain  Gain=2
  body_atti{,1..4} (5 alike) : Scope  NumInputPorts=2
  d : Gain  Gain=4
  p : Gain  Gain=10
  u : Outport
  wires:
  Sum3/1 -> body_atti3/1, Sum4/1
  1/b0/1 -> Sum4/2, body_atti2/2
  d/1 -> Sum3/2
  y/1 -> body_atti/2, LESO3/1(y)
  Sum2/1 -> d/1
  LESO3/3(z3) -> 1/b0/1
  p/1 -> Sum3/1
  LESO3/2(z2) -> body_atti4/1, Sum2/2
  Sum1/1 -> body_atti1/2, p/1
  b0/1 -> LESO3/2(b0u)
  LESO3/1(z1) -> body_atti/1, Sum1/2
  Sum4/1 -> body_atti3/2, u/1, b0/1
  des/1 -> Sum1/1
  Constant2/1 -> Sum2/1

== system freego_contact/Subsystem1/LADRC_Yaw ==
  des : Inport
  y : Inport  Port=2
  1/b0 : Gain  Gain=0.5
  Constant2 : Constant  Value=0
  LESO3 : Subsystem
  Sum1 : Sum  Inputs=|+-
  Sum2 : Sum  Inputs=|+-
  Sum3 : Sum  Inputs=+|+
  Sum4 : Sum  Inputs=|+-
  b0 : Gain  Gain=2
  body_atti : Scope  NumInputPorts=2
  body_atti1 : Scope  NumInputPorts=2
  body_atti2 : Scope  NumInputPorts=2
  d : Gain  Gain=4
  p : Gain  Gain=10
  u : Outport
  wires:
  Sum3/1 -> Sum4/1
  1/b0/1 -> Sum4/2, body_atti2/2
  d/1 -> Sum3/2
  y/1 -> body_atti/2, LESO3/1(y)
  Sum2/1 -> d/1
  LESO3/3(z3) -> 1/b0/1
  p/1 -> Sum3/1
  LESO3/2(z2) -> body_atti2/1, Sum2/2
  Sum1/1 -> p/1
  b0/1 -> LESO3/2(b0u)
  LESO3/1(z1) -> body_atti/1, Sum1/2
  Sum4/1 -> u/1, b0/1
  des/1 -> Sum1/1, body_atti1/1
  Constant2/1 -> Sum2/1, body_atti1/2

== system freego_contact/Subsystem/FLlegController/ab/ad_motorController ==
  pDes : Inport
  p : Inport  Port=2
  vDes : Inport  Port=3
  v : Inport  Port=4
  torDes : Inport  Port=5
  Kp : Inport  Port=6
  Kd : Inport  Port=7
  Product : Product
  Product1 : Product
  Sum1 : Sum  Inputs=|+-
  Sum2 : Sum  Inputs=|+-
  Sum3 : Sum  Inputs=+++
  torque : Outport
  wires:
  Sum1/1 -> Product1/1
  Product/1 -> Sum3/1
  vDes/1 -> Sum1/1
  v/1 -> Sum1/2
  p/1 -> Sum2/2
  Sum3/1 -> torque/1
  pDes/1 -> Sum2/1
  Sum2/1 -> Product/2
  Product1/1 -> Sum3/2
  torDes/1 -> Sum3/3
  Kp/1 -> Product/1
  Kd/1 -> Product1/2

== system freego_contact/Subsystem/FLlegController/hip_motorController ==
  pDes : Inport
  p : Inport  Port=2
  vDes : Inport  Port=3
  v : Inport  Port=4
  torDes : Inport  Port=5
  Kp : Inport  Port=6
  Kd : Inport  Port=7
  Product : Product
  Product1 : Product
  Sum1 : Sum  Inputs=|+-
  Sum2 : Sum  Inputs=|+-
  Sum3 : Sum  Inputs=+++
  torque : Outport
  wires:
  Sum1/1 -> Product1/1
  Product/1 -> Sum3/1
  vDes/1 -> Sum1/1
  v/1 -> Sum1/2
  p/1 -> Sum2/2
  Sum3/1 -> torque/1
  pDes/1 -> Sum2/1
  Sum2/1 -> Product/2
  Product1/1 -> Sum3/2
  torDes/1 -> Sum3/3
  Kp/1 -> Product/1
  Kd/1 -> Product1/2

== system freego_contact/Subsystem/FLlegController/knee_motorController ==
  pDes : Inport
  p : Inport  Port=2
  vDes : Inport  Port=3
  v : Inport  Port=4
  torDes : Inport  Port=5
  Kp : Inport  Port=6
  Kd : Inport  Port=7
  Product : Product
  Product1 : Product
  Sum1 : Sum  Inputs=|+-
  Sum2 : Sum  Inputs=|+-
  Sum3 : Sum  Inputs=+++
  torque : Outport
  wires:
  Sum1/1 -> Product1/1
  Product/1 -> Sum3/1
  vDes/1 -> Sum1/1
  v/1 -> Sum1/2
  p/1 -> Sum2/2
  Sum3/1 -> torque/1
  pDes/1 -> Sum2/1
  Sum2/1 -> Product/2
  Product1/1 -> Sum3/2
  torDes/1 -> Sum3/3
  Kp/1 -> Product/1
  Kd/1 -> Product1/2

== system freego_contact/Subsystem/FRlegController/ab/ad_motorController ==
  pDes : Inport
  p : Inport  Port=2
  vDes : Inport  Port=3
  v : Inport  Port=4
  torDes : Inport  Port=5
  Kp : Inport  Port=6
  Kd : Inport  Port=7
  Product : Product
  Product1 : Product
  Sum1 : Sum  Inputs=|+-
  Sum2 : Sum  Inputs=|+-
  Sum3 : Sum  Inputs=+++
  torque : Outport
  wires:
  Sum1/1 -> Product1/1
  Product/1 -> Sum3/1
  vDes/1 -> Sum1/1
  v/1 -> Sum1/2
  p/1 -> Sum2/2
  Sum3/1 -> torque/1
  pDes/1 -> Sum2/1
  Sum2/1 -> Product/2
  Product1/1 -> Sum3/2
  torDes/1 -> Sum3/3
  Kp/1 -> Product/1
  Kd/1 -> Product1/2

== system freego_contact/Subsystem/FRlegController/hip_motorController ==
  pDes : Inport
  p : Inport  Port=2
  vDes : Inport  Port=3
  v : Inport  Port=4
  torDes : Inport  Port=5
  Kp : Inport  Port=6
  Kd : Inport  Port=7
  Product : Product
  Product1 : Product
  Sum1 : Sum  Inputs=|+-
  Sum2 : Sum  Inputs=|+-
  Sum3 : Sum  Inputs=+++
  torque : Outport
  wires:
  Sum1/1 -> Product1/1
  Product/1 -> Sum3/1
  vDes/1 -> Sum1/1
  v/1 -> Sum1/2
  p/1 -> Sum2/2
  Sum3/1 -> torque/1
  pDes/1 -> Sum2/1
  Sum2/1 -> Product/2
  Product1/1 -> Sum3/2
  torDes/1 -> Sum3/3
  Kp/1 -> Product/1
  Kd/1 -> Product1/2

== system freego_contact/Subsystem/FRlegController/knee_motorController ==
  pDes : Inport
  p : Inport  Port=2
  vDes : Inport  Port=3
  v : Inport  Port=4
  torDes : Inport  Port=5
  Kp : Inport  Port=6
  Kd : Inport  Port=7
  Product : Product
  Product1 : Product
  Sum1 : Sum  Inputs=|+-
  Sum2 : Sum  Inputs=|+-
  Sum3 : Sum  Inputs=+++
  torque : Outport
  wires:
  Sum1/1 -> Product1/1
  Product/1 -> Sum3/1
  vDes/1 -> Sum1/1
  v/1 -> Sum1/2
  p/1 -> Sum2/2
  Sum3/1 -> torque/1
  pDes/1 -> Sum2/1
  Sum2/1 -> Product/2
  Product1/1 -> Sum3/2
  torDes/1 -> Sum3/3
  Kp/1 -> Product/1
  Kd/1 -> Product1/2

== system freego_contact/Subsystem/HLlegController/ab/ad_motorController ==
  pDes : Inport
  p : Inport  Port=2
  vDes : Inport  Port=3
  v : Inport  Port=4
  torDes : Inport  Port=5
  Kp : Inport  Port=6
  Kd : Inport  Port=7
  Product : Product
  Product1 : Product
  Sum1 : Sum  Inputs=|+-
  Sum2 : Sum  Inputs=|+-
  Sum3 : Sum  Inputs=+++
  torque : Outport
  wires:
  Sum1/1 -> Product1/1
  Product/1 -> Sum3/1
  vDes/1 -> Sum1/1
  v/1 -> Sum1/2
  p/1 -> Sum2/2
  Sum3/1 -> torque/1
  pDes/1 -> Sum2/1
  Sum2/1 -> Product/2
  Product1/1 -> Sum3/2
  torDes/1 -> Sum3/3
  Kp/1 -> Product/1
  Kd/1 -> Product1/2

== system freego_contact/Subsystem/HLlegController/hip_motorController ==
  pDes : Inport
  p : Inport  Port=2
  vDes : Inport  Port=3
  v : Inport  Port=4
  torDes : Inport  Port=5
  Kp : Inport  Port=6
  Kd : Inport  Port=7
  Product : Product
  Product1 : Product
  Sum1 : Sum  Inputs=|+-
  Sum2 : Sum  Inputs=|+-
  Sum3 : Sum  Inputs=+++
  torque : Outport
  wires:
  Sum1/1 -> Product1/1
  Product/1 -> Sum3/1
  vDes/1 -> Sum1/1
  v/1 -> Sum1/2
  p/1 -> Sum2/2
  Sum3/1 -> torque/1
  pDes/1 -> Sum2/1
  Sum2/1 -> Product/2
  Product1/1 -> Sum3/2
  torDes/1 -> Sum3/3
  Kp/1 -> Product/1
  Kd/1 -> Product1/2

== system freego_contact/Subsystem/HLlegController/knee_motorController ==
  pDes : Inport
  p : Inport  Port=2
  vDes : Inport  Port=3
  v : Inport  Port=4
  torDes : Inport  Port=5
  Kp : Inport  Port=6
  Kd : Inport  Port=7
  Product : Product
  Product1 : Product
  Sum1 : Sum  Inputs=|+-
  Sum2 : Sum  Inputs=|+-
  Sum3 : Sum  Inputs=+++
  torque : Outport
  wires:
  Sum1/1 -> Product1/1
  Product/1 -> Sum3/1
  vDes/1 -> Sum1/1
  v/1 -> Sum1/2
  p/1 -> Sum2/2
  Sum3/1 -> torque/1
  pDes/1 -> Sum2/1
  Sum2/1 -> Product/2
  Product1/1 -> Sum3/2
  torDes/1 -> Sum3/3
  Kp/1 -> Product/1
  Kd/1 -> Product1/2

== system freego_contact/Subsystem/HRlegController/ab/ad_motorController ==
  pDes : Inport
  p : Inport  Port=2
  vDes : Inport  Port=3
  v : Inport  Port=4
  torDes : Inport  Port=5
  Kp : Inport  Port=6
  Kd : Inport  Port=7
  Product : Product
  Product1 : Product
  Sum1 : Sum  Inputs=|+-
  Sum2 : Sum  Inputs=|+-
  Sum3 : Sum  Inputs=+++
  torque : Outport
  wires:
  Sum1/1 -> Product1/1
  Product/1 -> Sum3/1
  vDes/1 -> Sum1/1
  v/1 -> Sum1/2
  p/1 -> Sum2/2
  Sum3/1 -> torque/1
  pDes/1 -> Sum2/1
  Sum2/1 -> Product/2
  Product1/1 -> Sum3/2
  torDes/1 -> Sum3/3
  Kp/1 -> Product/1
  Kd/1 -> Product1/2

== system freego_contact/Subsystem/HRlegController/hip_motorController ==
  pDes : Inport
  p : Inport  Port=2
  vDes : Inport  Port=3
  v : Inport  Port=4
  torDes : Inport  Port=5
  Kp : Inport  Port=6
  Kd : Inport  Port=7
  Product : Product
  Product1 : Product
  Sum1 : Sum  Inputs=|+-
  Sum2 : Sum  Inputs=|+-
  Sum3 : Sum  Inputs=+++
  torque : Outport
  wires:
  Sum1/1 -> Product1/1
  Product/1 -> Sum3/1
  vDes/1 -> Sum1/1
  v/1 -> Sum1/2
  p/1 -> Sum2/2
  Sum3/1 -> torque/1
  pDes/1 -> Sum2/1
  Sum2/1 -> Product/2
  Product1/1 -> Sum3/2
  torDes/1 -> Sum3/3
  Kp/1 -> Product/1
  Kd/1 -> Product1/2

== system freego_contact/Subsystem/HRlegController/knee_motorController ==
  pDes : Inport
  p : Inport  Port=2
  vDes : Inport  Port=3
  v : Inport  Port=4
  torDes : Inport  Port=5
  Kp : Inport  Port=6
  Kd : Inport  Port=7
  Product : Product
  Product1 : Product
  Sum1 : Sum  Inputs=|+-
  Sum2 : Sum  Inputs=|+-
  Sum3 : Sum  Inputs=+++
  torque : Outport
  wires:
  Sum1/1 -> Product1/1
  Product/1 -> Sum3/1
  vDes/1 -> Sum1/1
  v/1 -> Sum1/2
  p/1 -> Sum2/2
  Sum3/1 -> torque/1
  pDes/1 -> Sum2/1
  Sum2/1 -> Product/2
  Product1/1 -> Sum3/2
  torDes/1 -> Sum3/3
  Kp/1 -> Product/1
  Kd/1 -> Product1/2

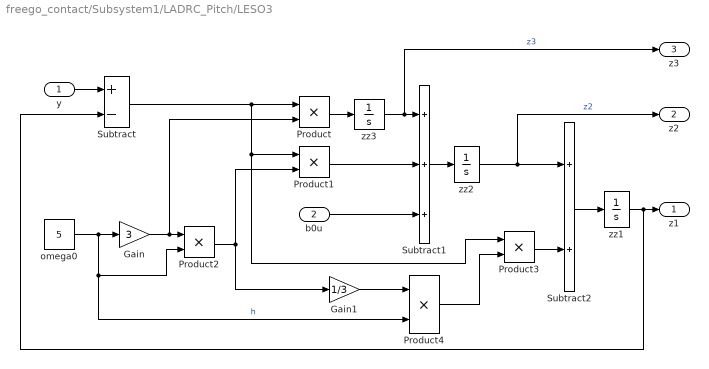
== system freego_contact/Subsystem1/LADRC_Pitch/LESO3 ==
  y : Inport
  b0u : Inport  Port=2
  Gain : Gain  Gain=3
  Gain1 : Gain  Gain=1/3
  Product{,1..4} (5 alike) : Product
  Subtract : Sum  Inputs=+-
  Subtract1 : Sum  Inputs=+++
  Subtract2 : Sum
  omega0 : Constant  Value=5
  zz1 : Integrator
  zz2 : Integrator
  zz3 : Integrator
  z1 : Outport
  z2 : Outport  Port=2
  z3 : Outport  Port=3
  wires:
  y/1 -> Subtract/1
  Subtract/1 -> Product/1, Product3/1, Product1/1
  omega0/1 -> Gain/1, Product4/2, Product2/2  "h"
  Gain/1 -> Product/2, Product2/1
  Product/1 -> zz3/1
  zz3/1 -> z3/1, Subtract1/1  "z3"
  b0u/1 -> Subtract1/3
  Product1/1 -> Subtract1/2
  Product2/1 -> Gain1/1, Product1/2
  Subtract1/1 -> zz2/1
  zz2/1 -> Subtract2/1, z2/1  "z2"
  zz1/1 -> Subtract/2, z1/1
  Product3/1 -> Subtract2/2
  Product4/1 -> Product3/2
  Subtract2/1 -> zz1/1
  Gain1/1 -> Product4/1

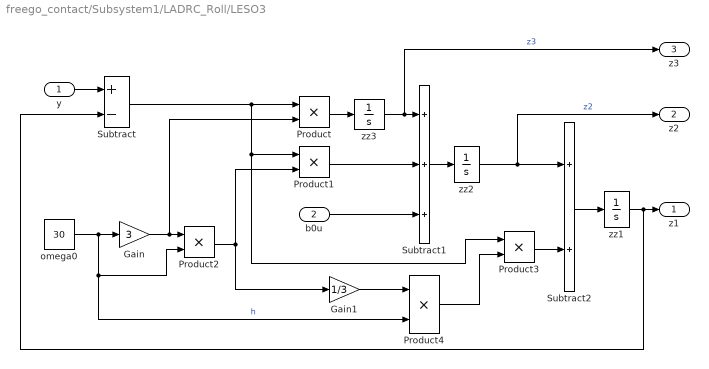
== system freego_contact/Subsystem1/LADRC_Roll/LESO3 ==
  y : Inport
  b0u : Inport  Port=2
  Gain : Gain  Gain=3
  Gain1 : Gain  Gain=1/3
  Product{,1..4} (5 alike) : Product
  Subtract : Sum  Inputs=+-
  Subtract1 : Sum  Inputs=+++
  Subtract2 : Sum
  omega0 : Constant  Value=30
  zz1 : Integrator
  zz2 : Integrator
  zz3 : Integrator
  z1 : Outport
  z2 : Outport  Port=2
  z3 : Outport  Port=3
  wires:
  y/1 -> Subtract/1
  Subtract/1 -> Product/1, Product3/1, Product1/1
  omega0/1 -> Gain/1, Product4/2, Product2/2  "h"
  Gain/1 -> Product/2, Product2/1
  Product/1 -> zz3/1
  zz3/1 -> z3/1, Subtract1/1  "z3"
  b0u/1 -> Subtract1/3
  Product1/1 -> Subtract1/2
  Product2/1 -> Gain1/1, Product1/2
  Subtract1/1 -> zz2/1
  zz2/1 -> Subtract2/1, z2/1  "z2"
  zz1/1 -> Subtract/2, z1/1
  Product3/1 -> Subtract2/2
  Product4/1 -> Product3/2
  Subtract2/1 -> zz1/1
  Gain1/1 -> Product4/1

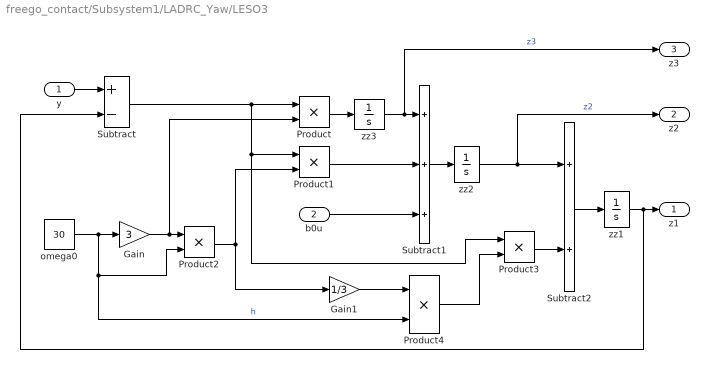
== system freego_contact/Subsystem1/LADRC_Yaw/LESO3 ==
  y : Inport
  b0u : Inport  Port=2
  Gain : Gain  Gain=3
  Gain1 : Gain  Gain=1/3
  Product{,1..4} (5 alike) : Product
  Subtract : Sum  Inputs=+-
  Subtract1 : Sum  Inputs=+++
  Subtract2 : Sum
  omega0 : Constant  Value=30
  zz1 : Integrator
  zz2 : Integrator
  zz3 : Integrator
  z1 : Outport
  z2 : Outport  Port=2
  z3 : Outport  Port=3
  wires:
  y/1 -> Subtract/1
  Subtract/1 -> Product/1, Product3/1, Product1/1
  omega0/1 -> Gain/1, Product4/2, Product2/2  "h"
  Gain/1 -> Product/2, Product2/1
  Product/1 -> zz3/1
  zz3/1 -> z3/1, Subtract1/1  "z3"
  b0u/1 -> Subtract1/3
  Product1/1 -> Subtract1/2
  Product2/1 -> Gain1/1, Product1/2
  Subtract1/1 -> zz2/1
  zz2/1 -> Subtract2/1, z2/1  "z2"
  zz1/1 -> Subtract/2, z1/1
  Product3/1 -> Subtract2/2
  Product4/1 -> Product3/2
  Subtract2/1 -> zz1/1
  Gain1/1 -> Product4/1

== matlab function TD/MATLAB Function1 ==
  data: x1 input double; fh output double; x2 input double; r input double; h input double
function  fh = fhan(x1, x2, r, h)
     d = r*h;
     d0 = h*d;
     y = x1 + h*x2;
     a0 = sqrt(d*d +8*r*abs(y));
     
     if abs(y)>d0
         a = x2 + (a0 - d)*sign(y)/2;
     else 
         a = x2 + y/h;
     end
     
     if abs(a)>d
         fh = -r*sign(a);
     else
         fh = -r*a/d;
     end
end

== matlab function LADRC/TD3 /MATLAB Function1 ==
  data: x1 input double; x2 input double; f output double; u input double; r input double; d input double
function f = fst2(x1, x2, u, r, d)
v=x1-u+abs(x2)*x2/(2*r);
if v>=d
    f=sign(v);
else f=v/d;
end

== matlab function Subsystem/FLlegController/MATLAB Function ==
  data: q input double; torque output double; sideSign input double; f_f input double; pDes input double; vDes input double; Kp input double; Kd input double
function torque = freegoCartesian(q, sideSign, f_f, pDes, vDes, Kp, Kd)
%FREEGO_JACOBIAN freego 腿部雅可比
torque = zeros(3,1); %关节转矩
footForce = zeros(3,1); %足端力

% global freego ;
% l1 = freego.abadLinkLength;
% l2 = freego.hipLinkLength;
% l3 = freego.kneeLinkLength;
% l4 = 0;
l1 = 0.062;
l2 = 0.209;
l3 = 0.195;
l4 = 0;

s1 = sin(q(1));
s2 = sin(q(2));
s3 = sin(q(3));

c1 = cos(q(1));
c2 = cos(q(2));
c3 = cos(q(3));

c23 = c2 * c3 - s2 * s3;
s23 = s2 * c3 + c2 * s3;

J = [0                                                          l3 * c23 + l2 * c2              l3 * c23;
    l3 * c1 * c23 + l2 * c1 * c2 - (l1+l4) * sideSign * s1     -l3 * s1 * s23 - l2 * s1 * s2   -l3 * s1 * s23;
    l3 * s1 * c23 + l2 * c2 * s1 + (l1+l4) * sideSign * c1      l3 * c1 * s23 + l2 * c1 * s2    l3 * c1 * s23];

P = [l3 * s23 + l2 * s2; (l1+l4) * sideSign * c1 + l3 * (s1 * c23) + l2 * c2 * s1; (l1+l4) * sideSign * s1 - l3 * (c1 * c23) - l2 * c1 * c2;];

V = J * q;

footForce(1) = f_f(1) + Kp(1)*(pDes(1) - P(1)) + Kd(1)*(vDes(1) - V(1));
footForce(2) = f_f(2) + Kp(2)*(pDes(2) - P(2)) + Kd(2)*(vDes(2) - V(2));
footForce(3) = f_f(3) + Kp(3)*(pDes(3) - P(3)) + Kd(3)*(vDes(3) - V(3));

torque = J' * footForce;

end

== matlab function Subsystem/FRlegController/MATLAB Function ==
  data: q input double; torque output double; sideSign input double; f_f input double; pDes input double; vDes input double; Kp input double; Kd input double
function torque = freegoCartesian(q, sideSign, f_f, pDes, vDes, Kp, Kd)
%FREEGO_JACOBIAN freego 腿部雅可比

torque = zeros(3,1); %关节转矩
footForce = zeros(3,1); %足端力

% global freego ;
% l1 = freego.abadLinkLength;
% l2 = freego.hipLinkLength;
% l3 = freego.kneeLinkLength;
% l4 = 0;
l1 = 0.062;
l2 = 0.209;
l3 = 0.195;
l4 = 0;

s1 = sin(q(1));
s2 = sin(q(2));
s3 = sin(q(3));

c1 = cos(q(1));
c2 = cos(q(2));
c3 = cos(q(3));

c23 = c2 * c3 - s2 * s3;
s23 = s2 * c3 + c2 * s3;

J = [0                                                          l3 * c23 + l2 * c2              l3 * c23;
    l3 * c1 * c23 + l2 * c1 * c2 - (l1+l4) * sideSign * s1     -l3 * s1 * s23 - l2 * s1 * s2   -l3 * s1 * s23;
    l3 * s1 * c23 + l2 * c2 * s1 + (l1+l4) * sideSign * c1      l3 * c1 * s23 + l2 * c1 * s2    l3 * c1 * s23];

P = [l3 * s23 + l2 * s2; (l1+l4) * sideSign * c1 + l3 * (s1 * c23) + l2 * c2 * s1; (l1+l4) * sideSign * s1 - l3 * (c1 * c23) - l2 * c1 * c2;];

V = J * q;

footForce(1) = f_f(1) + Kp(1)*(pDes(1) - P(1)) + Kd(1)*(vDes(1) - V(1));
footForce(2) = f_f(2) + Kp(2)*(pDes(2) - P(2)) + Kd(2)*(vDes(2) - V(2));
footForce(3) = f_f(3) + Kp(3)*(pDes(3) - P(3)) + Kd(3)*(vDes(3) - V(3));

torque = J' * footForce;

end

== matlab function Subsystem/HRlegController/MATLAB Function ==
  data: q input double; torque output double; sideSign input double; f_f input double; pDes input double; vDes input double; Kp input double; Kd input double
function torque = freegoCartesian(q, sideSign, f_f, pDes, vDes, Kp, Kd)
%FREEGO_JACOBIAN freego 腿部雅可比
torque = zeros(3,1); %关节转矩
footForce = zeros(3,1); %足端力

% global freego ;
% l1 = freego.abadLinkLength;
% l2 = freego.hipLinkLength;
% l3 = freego.kneeLinkLength;
% l4 = 0;
l1 = 0.062;
l2 = 0.209;
l3 = 0.195;
l4 = 0;

s1 = sin(q(1));
s2 = sin(q(2));
s3 = sin(q(3));

c1 = cos(q(1));
c2 = cos(q(2));
c3 = cos(q(3));

c23 = c2 * c3 - s2 * s3;
s23 = s2 * c3 + c2 * s3;

J = [0                                                          l3 * c23 + l2 * c2              l3 * c23;
    l3 * c1 * c23 + l2 * c1 * c2 - (l1+l4) * sideSign * s1     -l3 * s1 * s23 - l2 * s1 * s2   -l3 * s1 * s23;
    l3 * s1 * c23 + l2 * c2 * s1 + (l1+l4) * sideSign * c1      l3 * c1 * s23 + l2 * c1 * s2    l3 * c1 * s23];

P = [l3 * s23 + l2 * s2; (l1+l4) * sideSign * c1 + l3 * (s1 * c23) + l2 * c2 * s1; (l1+l4) * sideSign * s1 - l3 * (c1 * c23) - l2 * c1 * c2;];

V = J * q;

footForce(1) = f_f(1) + Kp(1)*(pDes(1) - P(1)) + Kd(1)*(vDes(1) - V(1));
footForce(2) = f_f(2) + Kp(2)*(pDes(2) - P(2)) + Kd(2)*(vDes(2) - V(2));
footForce(3) = f_f(3) + Kp(3)*(pDes(3) - P(3)) + Kd(3)*(vDes(3) - V(3));

torque = J' * footForce;

end

== matlab function Subsystem/HLlegController/MATLAB Function ==
  data: q input double; torque output double; sideSign input double; f_f input double; pDes input double; vDes input double; Kp input double; Kd input double
function torque = freegoCartesian(q, sideSign, f_f, pDes, vDes, Kp, Kd)
%FREEGO_JACOBIAN freego 腿部雅可比
torque = zeros(3,1); %关节转矩
footForce = zeros(3,1); %足端力

% global freego ;
% l1 = freego.abadLinkLength;
% l2 = freego.hipLinkLength;
% l3 = freego.kneeLinkLength;
% l4 = 0;
l1 = 0.062;
l2 = 0.209;
l3 = 0.195;
l4 = 0;

s1 = sin(q(1));
s2 = sin(q(2));
s3 = sin(q(3));

c1 = cos(q(1));
c2 = cos(q(2));
c3 = cos(q(3));

c23 = c2 * c3 - s2 * s3;
s23 = s2 * c3 + c2 * s3;

J = [0                                                          l3 * c23 + l2 * c2              l3 * c23;
    l3 * c1 * c23 + l2 * c1 * c2 - (l1+l4) * sideSign * s1     -l3 * s1 * s23 - l2 * s1 * s2   -l3 * s1 * s23;
    l3 * s1 * c23 + l2 * c2 * s1 + (l1+l4) * sideSign * c1      l3 * c1 * s23 + l2 * c1 * s2    l3 * c1 * s23];

P = [l3 * s23 + l2 * s2; (l1+l4) * sideSign * c1 + l3 * (s1 * c23) + l2 * c2 * s1; (l1+l4) * sideSign * s1 - l3 * (c1 * c23) - l2 * c1 * c2;];

V = J * q;

footForce(1) = f_f(1) + Kp(1)*(pDes(1) - P(1)) + Kd(1)*(vDes(1) - V(1));
footForce(2) = f_f(2) + Kp(2)*(pDes(2) - P(2)) + Kd(2)*(vDes(2) - V(2));
footForce(3) = f_f(3) + Kp(3)*(pDes(3) - P(3)) + Kd(3)*(vDes(3) - V(3));

torque = J' * footForce;

end
